simulink model "Hierarchy3"  (Simulink 5.0)
settings: Solver=ode45  StartTime=0.0  StopTime=10.0  RelTol=1e-3
settings Model: Creator=scaife  LastModifiedBy=scaife  ExtModeAutoUpdateStatusClock=off

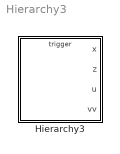
== system Hierarchy3 ==
  Hierarchy3 : Stateflow chart

== stateflow chart Hierarchy3 ==
  state TOP1 [parallel]
    state A
      state A1/
        en: x=0
      state A2/
        en: x=5
      A1 -> (junction 17) : E[x<5]{y=1}
      (junction 17) -> A2 : [x>=5]
      A2 -> (junction 18) : E[x>0]{y=-1}
      (junction 18) -> A1 : [x<=0]
      (default) -> A1
      (junction 17) -> (junction 18) : {x+=y}
      (junction 18) -> (junction 17) : {x+=y}
    state B
      state B1/
        en: z=0
      state B2/
        en: z=5
      (junction 19) -> B1 : [z<=0]
      (default) -> B1
      B2 -> (junction 19) : E[z>0]{y=-1}
      (junction 19) -> (junction 20) : {z+=y}
      (junction 20) -> (junction 19) : {z+=y}
      B1 -> (junction 20) : E[z<5]{y=1}
      (junction 20) -> B2 : [z>=5]
    (default) -> A
    A -> (junction 21) : F{i=0}
    (junction 21) -> B
    B -> (junction 22) : F{i=3}
    (junction 22) -> A
    (junction 21) -> (junction 21) : [i<3]{i++}
    (junction 22) -> (junction 22) : [i>0]{i--}
  state TOP2 [parallel]
    state C
      state C1/
        en: vv=0
      state C2/
        en:vv=5
      (junction 25) -> C1 : [vv<=0]
      (default) -> C1
      C2 -> (junction 25) : E[vv>0]{w=-1}
      (junction 25) -> (junction 26) : {vv+=w}
      (junction 26) -> (junction 25) : {vv+=w}
      C1 -> (junction 26) : E[vv<5]{w=1}
      (junction 26) -> C2 : [vv>=5]
    state D
      state D1/
        en: u=0
      state D2/
        en: u=5
      (junction 27) -> D1 : [u<=0]
      (default) -> D1
      D2 -> (junction 27) : E[u>0]{w=-1}
      (junction 27) -> (junction 28) : {u+=w}
      (junction 28) -> (junction 27) : {u+=w}
      D1 -> (junction 28) : E[u<5]{w=1}
      (junction 28) -> D2 : [u>=5]
    (default) -> C
    (junction 23) -> C
    C -> (junction 24) : F{j=0}
    (junction 23) -> (junction 23) : [j>0]{j--}
    D -> (junction 23) : F{j=3}
    (junction 24) -> (junction 24) : [j<3]{j++}
    (junction 24) -> D
  data: y local int32; x output int32; z output int32; i local int32; j local int32; w local int32; u output int32; vv output int32
  events: E input EITHER_EDGE_EVENT; F input EITHER_EDGE_EVENT
